simulink model "bai2"  (R2017b)
settings: Solver=ode4  StartTime=0.0  StopTime=20  FixedStep=0.01  RelTol=1e-3
libraries: fuzblock x1
settings Model: Creator=DELL  LastModifiedBy=phamt

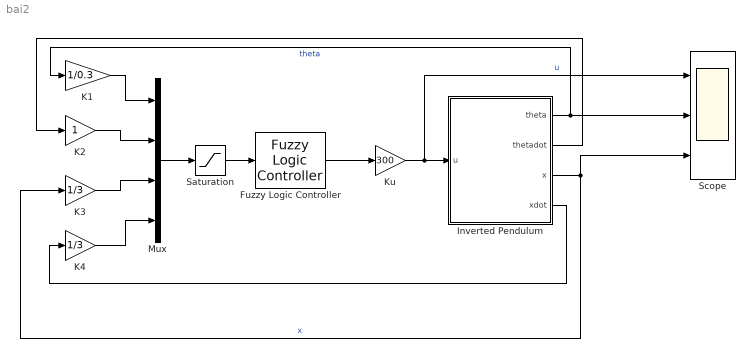
== system bai2 ==
  Fuzzy Logic Controller : fuzblock/Fuzzy Logic  Controller  FIS='bai2_FIS.fis'  OutputSampleNumber=101  DataType=double  FuzzifiedInputs=off  RuleFiringStrengths=off  RuleOutputs=off  AggregatedOutputs=off  SimulateUsing=Interpreted execution
  Inverted Pendulum : Subsystem  mask{M=5, n=3, l=1, g=9.81, x0=3, xdot0=-2, theta0=0.2, thetadot0=-1}
      mask prompts: M "trong luong xe"; n "trong luong con lac"; l "chieu dai con lac"; g "gia toc trong truong"; x0 "vi tri xe ban dau"; xdot0 "van toc xe ban dau"; theta0 "goc ban dau"; thetadot0 "van toc goc ban dau"
  "K1 " : Gain  Gain=1/0.3
  "K2 " : Gain
  "K3 " : Gain  Gain=1/3
  "K4 " : Gain  Gain=1/3
  Ku : Gain  Gain=300
  Mux : Mux
  Saturation : Saturate  UpperLimit=1  LowerLimit=-1
  Scope : Scope  NumInputPorts=3
  wires:
  Ku/1 -> Scope/1, Inverted Pendulum/1(u)  "u"
  Fuzzy Logic Controller/1 -> Ku/1
  Saturation/1 -> Fuzzy Logic Controller/1
  Mux/1 -> Saturation/1
  "K1 "/1 -> Mux/1
  "K2 "/1 -> Mux/2
  "K3 "/1 -> Mux/3
  "K4 "/1 -> Mux/4
  Inverted Pendulum/1(theta) -> "K1 "/1, Scope/2  "theta"
  Inverted Pendulum/2(thetadot) -> "K2 "/1
  Inverted Pendulum/4(xdot) -> "K4 "/1
  Inverted Pendulum/3(x) -> Scope/3, "K3 "/1  "x"

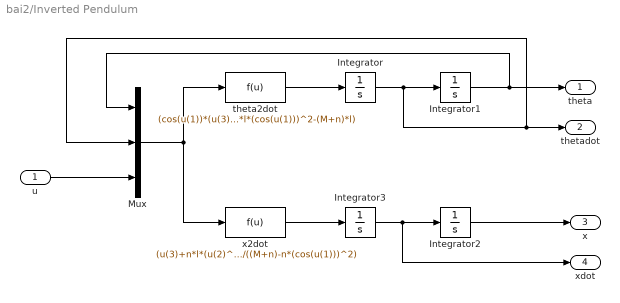
== system bai2/Inverted Pendulum ==
  u : Inport
  Integrator : Integrator  InitialCondition=thetadot0
  Integrator1 : Integrator  InitialCondition=theta0
  Integrator2 : Integrator  InitialCondition=x0
  Integrator3 : Integrator  InitialCondition=xdot0
  Mux : Mux  Inputs=3
  theta2dot : Fcn  Expr=(cos(u(1))*(u(3)+n*l*(u(2))^2*sin(u(1)))-(M+n)*(g*sin(u(1))))/(n*l*(cos(u(1)))^2-(M+n)*l)
  x2dot : Fcn  Expr=(u(3)+n*l*(u(2)^2)*sin(u(1))-n*g*sin(u(1))*cos(u(1)))/((M+n)-n*(cos(u(1)))^2)
  theta : Outport
  thetadot : Outport  Port=2
  x : Outport  Port=3
  xdot : Outport  Port=4
  wires:
  theta2dot/1 -> Integrator/1
  Integrator/1 -> Mux/2, thetadot/1, Integrator1/1
  x2dot/1 -> Integrator3/1
  Integrator3/1 -> xdot/1, Integrator2/1
  Integrator1/1 -> Mux/1, theta/1
  Integrator2/1 -> x/1
  Mux/1 -> x2dot/1, theta2dot/1
  u/1 -> Mux/3
